simulink model "Simulacion_caminata"  (R2023a)
settings: Solver=VariableStepAuto  StartTime=0.0  StopTime=3  RelTol=1e-3
undefined symbols (not defined in the file): alfa_inicial, d, r1, vel_caminata
settings Model: Creator=tobip  LastModifiedBy=tobip

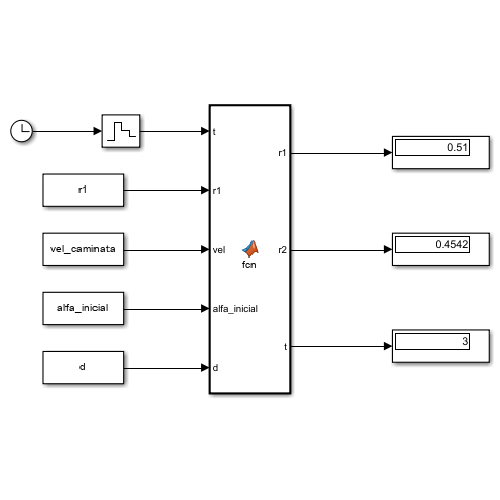
[thumbnail: Simulink's stored preview of the top-level diagram]
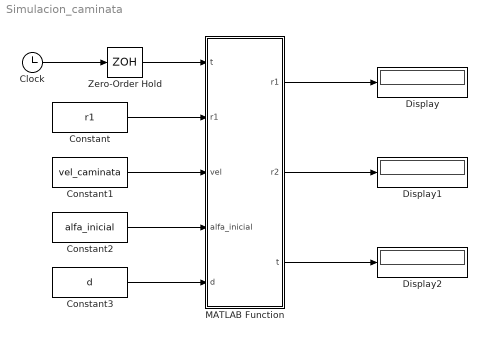
== system Simulacion_caminata ==
  Clock : Clock
  Constant : Constant  Value=r1
  Constant1 : Constant  Value=vel_caminata
  Constant2 : Constant  Value=alfa_inicial
  Constant3 : Constant  Value=d
  Display : Display
  Display1 : Display
  Display2 : Display
  MATLAB Function : MATLAB Function  TreatAsAtomicUnit=on
  Zero-Order Hold : ZeroOrderHold  SampleTime=0.1
  wires:
  Clock/1 -> Zero-Order Hold/1
  Constant/1 -> MATLAB Function/2("r1 ")
  Constant1/1 -> MATLAB Function/3(vel)
  Constant2/1 -> MATLAB Function/4(alfa_inicial)
  Constant3/1 -> MATLAB Function/5(d)
  MATLAB Function/1(r1) -> Display/1
  MATLAB Function/2(r2) -> Display1/1
  MATLAB Function/3(t) -> Display2/1
  Zero-Order Hold/1 -> MATLAB Function/1("t ")

== matlab function Simulacion_caminata/MATLAB Function ==
  data: t input; r1 output; r1 input; vel input; alfa_inicial input; d input; r2 output; t output
function [r1, r2,t] = fcn(t, r1, vel, alfa_inicial, d)

persistent h fig

omega = vel/r1;
alfa = alfa_inicial + omega*t;
r2 = sqrt((r1^2) + (d^2) - 2*r1*d*cos(alfa));   %Distancia a mic2

x1 = r1*cos(alfa);
y1 = r1*sin(alfa);

% Inicializar el gráfico
if isempty(h)
    fig = figure('Name', 'Caminata en el plano', 'NumberTitle', 'off');
    h = plot(0, 0, 'ro', 'MarkerSize', 10, 'MarkerFaceColor', 'r');
    axis([-1 1 -1 1]); % Ajusta los límites según el rango de tu simulación
    grid on;
    xlabel('X (m)');
    ylabel('Y (m)');
    title('Caminata en el plano');
end

% Actualizar el punto
if ishandle(h)  % Cambiado de 'isvalid' a 'ishandle'
    set(h, 'XData', x1, 'YData', y1);
    hold on
     plot(d/2, 0, 'ro' ,'MarkerSize', 30, 'MarkerFaceColor', 'k');
    plot(0, 0, 'ro' ,'MarkerSize', 4, 'MarkerFaceColor', 'b');
    plot(d, 0, 'ro' ,'MarkerSize', 4, 'MarkerFaceColor', 'b');
    hold off
    drawnow;
end
end
